simulink model "NGV_2_2"  (R2022b)
settings: Solver=VariableStepAuto  StartTime=0.0  StopTime=100  RelTol=1e-3
model workspace (MAT data in the model file):
  B = 1
  J = 1
  Ke = 1
  Ki = 1
  Kp = 1
  Kt = 1
  L = 1
  R = 1
libraries: pil_lib x1
settings Model: Creator=user  LastModifiedBy=123
settings SolverCC: AlgebraicLoopSolver=TrustRegion
settings OptimizationCC: ReuseModelBlockBuffer=on
settings DebuggingCC: UnconnectedInputMsg=warning  UnconnectedOutputMsg=warning  UnconnectedLineMsg=warning
settings ModelReferenceCC: EnableRefExpFcnMdlSchedulingChecks=on
settings RTWCC: DLArmComputeVersion=19.05

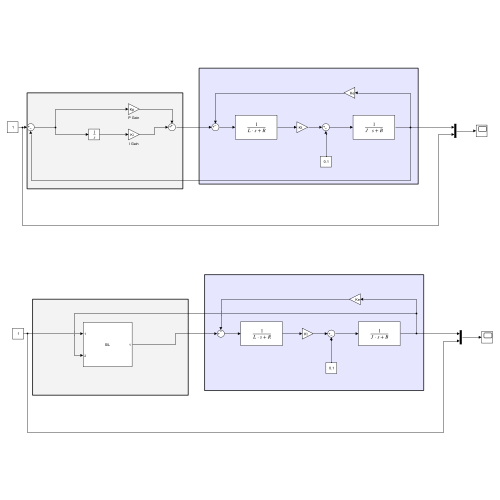
[thumbnail: Simulink's stored preview of the top-level diagram]
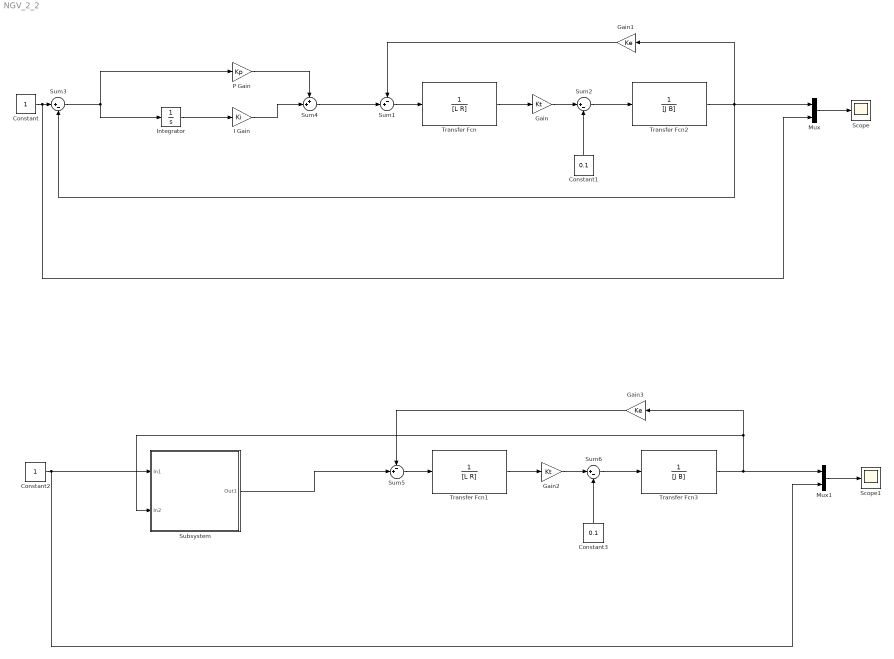
== system NGV_2_2 ==
  Constant : Constant
  Constant1 : Constant  Value=0.1
  Constant2 : Constant
  Constant3 : Constant  Value=0.1
  Gain : Gain  Gain=Kt
  Gain1 : Gain  Gain=Ke
  Gain2 : Gain  Gain=Kt
  Gain3 : Gain  Gain=Ke
  I Gain : Gain  Gain=Ki
  Integrator : Integrator
  Mux : Mux  Inputs=2
  Mux1 : Mux  Inputs=2
  P Gain : Gain  Gain=Kp
  Scope : Scope
  Scope1 : Scope
  Subsystem : Subsystem  Tag=__SL_testing_harness_stub_  DialogController=pil_create_dialog  LoadFcn=|
      | try
      |    if ~strcmp(rtw.pil.getPILVersion, '9.14 (R2023a)_15')
      |       set_param(gcb, 'DialogController', '');
      |       set_param(gcb, 'DialogControllerArgs', '');
      |    end
      | catch e
      |       set_param(gcb, 'DialogController', '');
      |       set_param(gcb, 'DialogControllerArgs', '');
      | end
      mask help: PIL:pil:XILBlockMaskDesc
      mask Display: disp('SIL');
  Sum1 : Sum  Inputs=-+|
  Sum2 : Sum  Inputs=|+-
  Sum3 : Sum  Inputs=|+-
  Sum4 : Sum  Inputs=++|
  Sum5 : Sum  Inputs=-+|
  Sum6 : Sum  Inputs=|+-
  Transfer Fcn : TransferFcn  Denominator=[L R]
  Transfer Fcn1 : TransferFcn  Denominator=[L R]
  Transfer Fcn2 : TransferFcn  Denominator=[J B]
  Transfer Fcn3 : TransferFcn  Denominator=[J B]
  wires:
  Transfer Fcn/1 -> Gain/1
  Sum1/1 -> Transfer Fcn/1
  Sum2/1 -> Transfer Fcn2/1
  Transfer Fcn2/1 -> Mux/1, Sum3/2, Gain1/1
  Gain1/1 -> Sum1/1
  Gain/1 -> Sum2/1
  Sum3/1 -> P Gain/1, Integrator/1
  Constant/1 -> Mux/2, Sum3/1
  Mux/1 -> Scope/1
  Constant1/1 -> Sum2/2
  Sum4/1 -> Sum1/2
  Integrator/1 -> I Gain/1
  I Gain/1 -> Sum4/2
  P Gain/1 -> Sum4/1
  Transfer Fcn1/1 -> Gain2/1
  Sum5/1 -> Transfer Fcn1/1
  Subsystem/1(Out1) -> Sum5/2
  Gain2/1 -> Sum6/1
  Constant3/1 -> Sum6/2
  Gain3/1 -> Sum5/1
  Constant2/1 -> Subsystem/1(In1), Mux1/2
  Sum6/1 -> Transfer Fcn3/1
  Transfer Fcn3/1 -> Subsystem/2(In2), Gain3/1, Mux1/1
  Mux1/1 -> Scope1/1

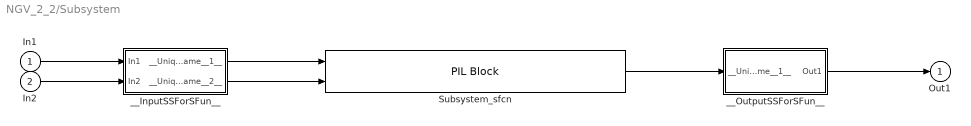
== system NGV_2_2/Subsystem ==
  In1 : Inport
  In2 : Inport  Port=2
  Subsystem_sfcn : pil_lib/PIL Block  SimulationMode=SIL  IsTopModelPIL=off  CodeDir=Subsystem_ert_rtw  AnchorDir=C:\Users\123\Desktop\bearing  ConfigName=Software-in-the-Loop (SIL)  XrelIsTopModelCode=on  XrelIsReusable=off  XrelDWorkNames={}  XrelDWorkTypes={}  XrelModelArgVals={}  XrelOrderedParamNames={}
  __InputSSForSFun__ : Subsystem
  __OutputSSForSFun__ : Subsystem
  Out1 : Outport
  wires:
  __OutputSSForSFun__/1(Out1) -> Out1/1
  Subsystem_sfcn/1 -> __OutputSSForSFun__/1(__UniqueInportName__1__)
  __InputSSForSFun__/2(__UniqueOutportName__2__) -> Subsystem_sfcn/2
  __InputSSForSFun__/1(__UniqueOutportName__1__) -> Subsystem_sfcn/1
  In2/1 -> __InputSSForSFun__/2(In2)
  In1/1 -> __InputSSForSFun__/1(In1)

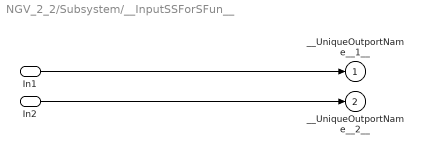
== system NGV_2_2/Subsystem/__InputSSForSFun__ ==
  In1 : Inport
  In2 : Inport  Port=2
  __UniqueOutportName__1__ : Outport
  __UniqueOutportName__2__ : Outport  Port=2
  wires:
  In2/1 -> __UniqueOutportName__2__/1
  In1/1 -> __UniqueOutportName__1__/1

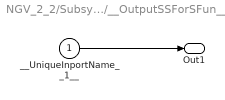
== system NGV_2_2/Subsystem/__OutputSSForSFun__ ==
  __UniqueInportName__1__ : Inport
  Out1 : Outport
  wires:
  __UniqueInportName__1__/1 -> Out1/1
